simulink model "Car_State"  (R2023b)
settings: Solver=FixedStepAuto  StartTime=0.0  StopTime=10.0  RelTol=1e-3
libraries: simulink x5
settings Model: Creator=cspt  LastModifiedBy=joser
settings SolverCC: AlgebraicLoopSolver=TrustRegion
settings DataIOCC: SaveOutput=off  ReturnWorkspaceOutputs=off
settings OptimizationCC: DefaultParameterBehavior=Inlined
settings DebuggingCC: UnconnectedInputMsg=warning  UnconnectedOutputMsg=warning  UnconnectedLineMsg=warning  ArithmeticOperatorsInVariantConditions=warning
settings ModelReferenceCC: EnableRefExpFcnMdlSchedulingChecks=on
settings SFSimCC: SimUseLocalCustomCode=off  CustomCodeUndefinedFunction=UseInterfaceOnly
settings RTWCC: Description=INTECRIO Real-Time Target  SystemTargetFile=irt.tlc  TemplateMakefile=irt_default_tmf  RTWUseLocalCustomCode=off
settings STFCustomTargetCC: UtilityFuncGeneration=Shared location  MatFileLogging=on  GRTInterface=on  SystemTargetFile=irt.tlc
settings GRTTargetCC: UtilityFuncGeneration=Shared location  ParMdlRefBuildCompliant=off  CompOptLevelCompliant=off  ConcurrentExecutionCompliant=off  CombineOutputUpdateFcns=off  CPPClassGenCompliant=off  GRTInterface=on  UseToolchainInfoCompliant=off  GenerateASAP2=on

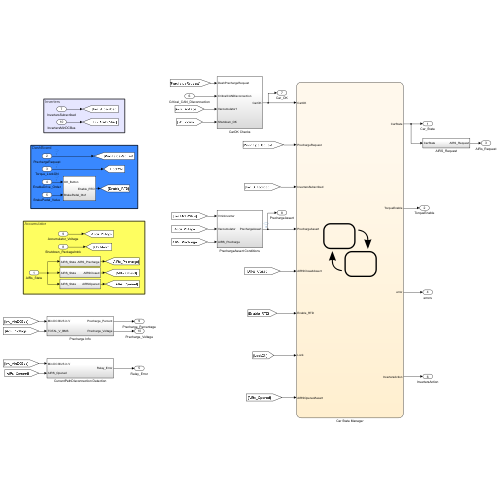
[thumbnail: Simulink's stored preview of the top-level diagram]
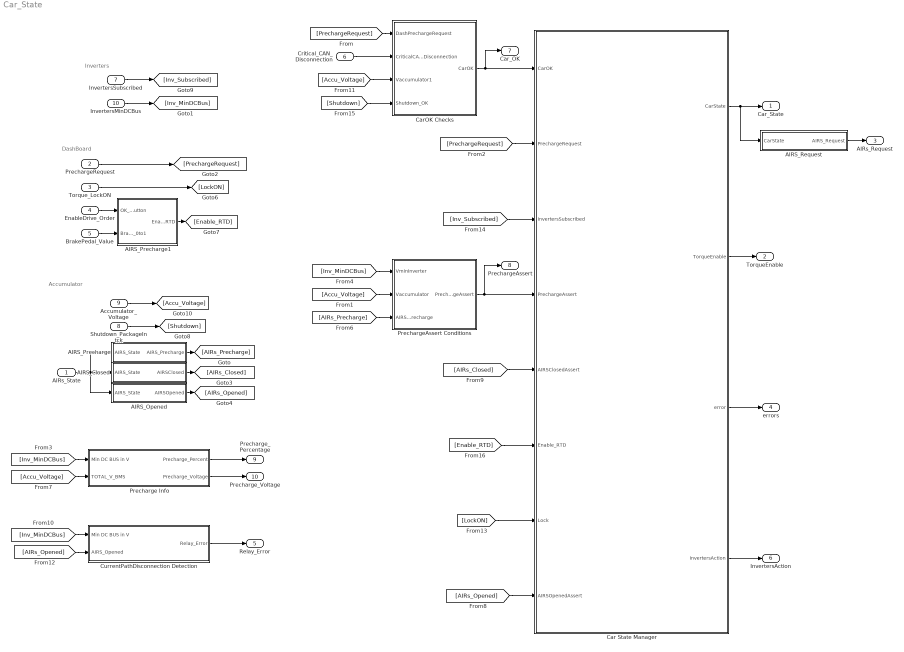
== system Car_State ==
  note: DashBoard
  note: Accumulator
  note: Inverters
  AIRs_State : Inport
  PrechargeRequest : Inport  Port=2
  Torque_LockON : Inport  Port=3
  EnableDrive_Order : Inport  Port=4
  BrakePedal_Value : Inport  Port=5
  Critical_CAN_Disconnection : Inport  Port=6
  InvertersSubscribed : Inport  Port=7
  Shutdown_PackageIntck : Inport  Port=8
  Accumulator_Voltage : Inport  Port=9  OutDataTypeStr=double  Unit=V
  InvertersMinDCBus : Inport  Port=10  Unit=V
  AIRS_Closed : Subsystem
  AIRS_Opened : Subsystem
  AIRS_Precharge : Subsystem
  AIRS_Precharge1 : Subsystem
  AIRS_Request : Subsystem
  Car State Manager : Stateflow chart  TreatAsAtomicUnit=on  SystemSampleTime=0.025
  CarOK Checks : Subsystem
  CurrentPathDisconnection Detection : Subsystem
  Precharge Info : Subsystem
  PrechargeAssert Conditions : Subsystem
  Car_State : Outport  VectorParamsAs1DForOutWhenUnconnected=off
  TorqueEnable : Outport  Port=2  VectorParamsAs1DForOutWhenUnconnected=off
  AIRs_Request : Outport  Port=3  VectorParamsAs1DForOutWhenUnconnected=off
  errors : Outport  Port=4  VectorParamsAs1DForOutWhenUnconnected=off
  Relay_Error : Outport  Port=5  VectorParamsAs1DForOutWhenUnconnected=off
  InvertersAction : Outport  Port=6  VectorParamsAs1DForOutWhenUnconnected=off
  Car_OK : Outport  Port=7  VectorParamsAs1DForOutWhenUnconnected=off
  PrechargeAssert : Outport  Port=8  VectorParamsAs1DForOutWhenUnconnected=off
  Precharge_Percentage : Outport  Port=9  VectorParamsAs1DForOutWhenUnconnected=off
  Precharge_Voltage : Outport  Port=10  VectorParamsAs1DForOutWhenUnconnected=off
  wires:
  CurrentPathDisconnection Detection/1(Relay_Error) -> Relay_Error/1
  Car State Manager/1(CarState) -> AIRS_Request/1(CarState), Car_State/1
  [PrechargeRequest] -> CarOK Checks/1(DashPrechargeRequest)
  AIRS_Request/1(AIRS_Request) -> AIRs_Request/1
  Car State Manager/4(InvertersAction) -> InvertersAction/1
  Car State Manager/2(TorqueEnable) -> TorqueEnable/1
  Car State Manager/3(error) -> errors/1
  CarOK Checks/1(CarOK) -> Car_OK/1, Car State Manager/1(CarOK)
  PrechargeRequest/1 -> [PrechargeRequest]
  AIRs_State/1 -> AIRS_Opened/1(AIRS_State), AIRS_Precharge/1(AIRS_State), AIRS_Closed/1(AIRS_State)
  Critical_CAN_Disconnection/1 -> CarOK Checks/2(CriticalCANDisconnection)
  Shutdown_PackageIntck/1 -> [Shutdown]
  [PrechargeRequest] -> Car State Manager/2(PrechargeRequest)
  [AIRs_Opened] -> Car State Manager/8(AIRSOpenedAssert)
  [AIRs_Closed] -> Car State Manager/5(AIRSClosedAssert)
  Torque_LockON/1 -> [LockON]
  EnableDrive_Order/1 -> AIRS_Precharge1/1(OK_Button)
  [Enable_RTD] -> Car State Manager/6(Enable_RTD)
  [LockON] -> Car State Manager/7(Lock)
  InvertersSubscribed/1 -> [Inv_Subscribed]
  [Inv_Subscribed] -> Car State Manager/3(InvertersSubscribed)
  [Shutdown] -> CarOK Checks/4(Shutdown_OK)
  PrechargeAssert Conditions/1(PrechargeAssert) -> Car State Manager/4(PrechargeAssert), PrechargeAssert/1
  [Inv_MinDCBus] -> Precharge Info/1(Min DC BUS in V)
  Precharge Info/1(Precharge_Percent) -> Precharge_Percentage/1
  Precharge Info/2(Precharge_Voltage) -> Precharge_Voltage/1
  [Inv_MinDCBus] -> CurrentPathDisconnection Detection/1(Min DC BUS in V)
  [AIRs_Opened] -> CurrentPathDisconnection Detection/2(AIRS_Opened)
  [Accu_Voltage] -> PrechargeAssert Conditions/2(Vaccumulator)
  [Inv_MinDCBus] -> PrechargeAssert Conditions/1(VminInverter)
  [AIRs_Precharge] -> PrechargeAssert Conditions/3(AIRS_Precharge)
  [Accu_Voltage] -> Precharge Info/2(TOTAL_V_BMS)
  Accumulator_Voltage/1 -> [Accu_Voltage]
  InvertersMinDCBus/1 -> [Inv_MinDCBus]
  AIRS_Closed/1(AIRSClosed) -> [AIRs_Closed]
  [Accu_Voltage] -> CarOK Checks/3(Vaccumulator1)
  AIRS_Precharge/1(AIRS_Precharge) -> [AIRs_Precharge]
  AIRS_Opened/1(AIRSOpened) -> [AIRs_Opened]
  BrakePedal_Value/1 -> AIRS_Precharge1/2(BrakePedal_0to1)
  AIRS_Precharge1/1(Enable_RTD) -> [Enable_RTD]

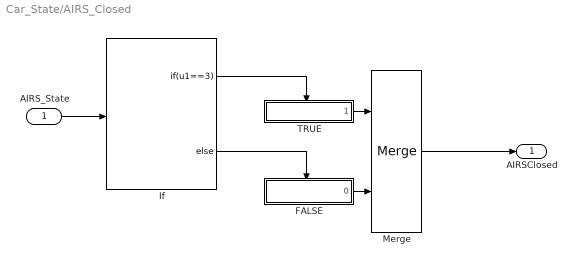
== system Car_State/AIRS_Closed ==
  AIRS_State : Inport
  FALSE : Subsystem  TreatAsAtomicUnit=on
  If : If  IfExpression=u1==3
  Merge : Merge
  TRUE : Subsystem  TreatAsAtomicUnit=on
  AIRSClosed : Outport  VectorParamsAs1DForOutWhenUnconnected=off
  wires:
  Merge/1 -> AIRSClosed/1
  FALSE/1(0) -> Merge/2
  If/2 -> FALSE/Action
  TRUE/1(1) -> Merge/1
  If/1 -> TRUE/Action
  AIRS_State/1 -> If/1

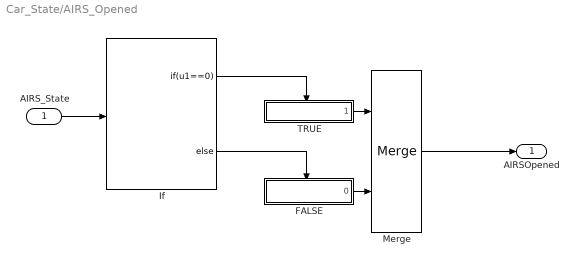
== system Car_State/AIRS_Opened ==
  AIRS_State : Inport
  FALSE : Subsystem  TreatAsAtomicUnit=on
  If : If  IfExpression=u1==0
  Merge : Merge
  TRUE : Subsystem  TreatAsAtomicUnit=on
  AIRSOpened : Outport  VectorParamsAs1DForOutWhenUnconnected=off
  wires:
  Merge/1 -> AIRSOpened/1
  FALSE/1(0) -> Merge/2
  If/2 -> FALSE/Action
  TRUE/1(1) -> Merge/1
  If/1 -> TRUE/Action
  AIRS_State/1 -> If/1

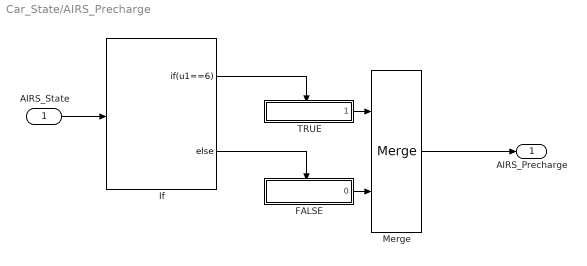
== system Car_State/AIRS_Precharge ==
  AIRS_State : Inport
  FALSE : Subsystem  TreatAsAtomicUnit=on
  If : If  IfExpression=u1==6
  Merge : Merge
  TRUE : Subsystem  TreatAsAtomicUnit=on
  AIRS_Precharge : Outport  VectorParamsAs1DForOutWhenUnconnected=off
  wires:
  Merge/1 -> AIRS_Precharge/1
  FALSE/1(0) -> Merge/2
  If/2 -> FALSE/Action
  TRUE/1(1) -> Merge/1
  If/1 -> TRUE/Action
  AIRS_State/1 -> If/1

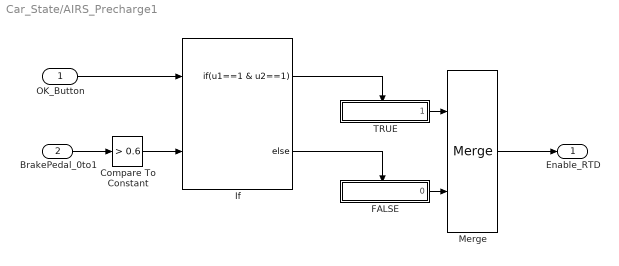
== system Car_State/AIRS_Precharge1 ==
  OK_Button : Inport
  BrakePedal_0to1 : Inport  Port=2
  Compare To Constant : simulink/Logic and Bit Operations/Compare To Constant  relop=>  const=0.6  OutDataTypeStr=boolean
  FALSE : Subsystem  TreatAsAtomicUnit=on
  If : If  NumInputs=2  IfExpression=u1==1 & u2==1
  Merge : Merge
  TRUE : Subsystem  TreatAsAtomicUnit=on
  Enable_RTD : Outport  VectorParamsAs1DForOutWhenUnconnected=off
  wires:
  Merge/1 -> Enable_RTD/1
  FALSE/1(0) -> Merge/2
  If/2 -> FALSE/Action
  TRUE/1(1) -> Merge/1
  If/1 -> TRUE/Action
  OK_Button/1 -> If/1
  BrakePedal_0to1/1 -> Compare To Constant/1
  Compare To Constant/1 -> If/2

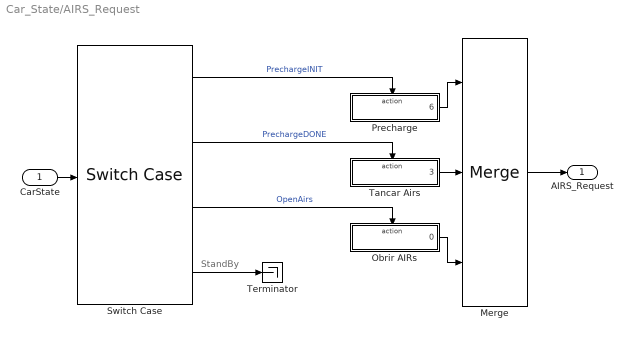
== system Car_State/AIRS_Request ==
  note: StandBy
  CarState : Inport
  Merge : Merge  Inputs=3
  Obrir AIRs : Subsystem  TreatAsAtomicUnit=on
  Precharge : Subsystem  TreatAsAtomicUnit=on
  Switch Case : SwitchCase  CaseConditions={6,9,21}
  Tancar Airs : Subsystem  TreatAsAtomicUnit=on
  Terminator : Terminator
  AIRS_Request : Outport  VectorParamsAs1DForOutWhenUnconnected=off
  wires:
  Merge/1 -> AIRS_Request/1
  Switch Case/2 -> Tancar Airs/Action  "PrechargeDONE"
  Switch Case/1 -> Precharge/Action  "PrechargeINIT"
  CarState/1 -> Switch Case/1
  Switch Case/3 -> Obrir AIRs/Action  "OpenAirs"
  Precharge/1(6) -> Merge/1
  Tancar Airs/1(3) -> Merge/2
  Obrir AIRs/1(0) -> Merge/3
  Switch Case/4 -> Terminator/1

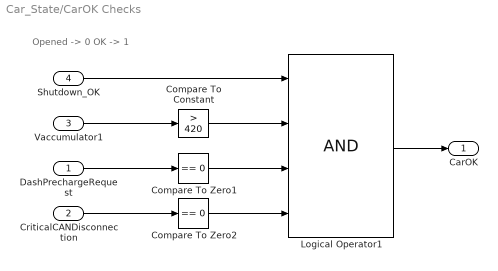
== system Car_State/CarOK Checks ==
  note: Opened -> 0
      | OK -> 1
  DashPrechargeRequest : Inport
  CriticalCANDisconnection : Inport  Port=2
  Vaccumulator1 : Inport  Port=3
  Shutdown_OK : Inport  Port=4
  Compare To Constant : simulink/Logic and Bit Operations/Compare To Constant  relop=>  const=420  OutDataTypeStr=boolean
  Compare To Zero1 : simulink/Logic and Bit Operations/Compare To Zero  relop===  OutDataTypeStr=boolean
  Compare To Zero2 : simulink/Logic and Bit Operations/Compare To Zero  relop===  OutDataTypeStr=boolean
  Logical Operator1 : Logic  Inputs=4  AllPortsSameDT=off  OutDataTypeStr=boolean
  CarOK : Outport  VectorParamsAs1DForOutWhenUnconnected=off
  wires:
  Logical Operator1/1 -> CarOK/1
  DashPrechargeRequest/1 -> Compare To Zero1/1
  Compare To Zero1/1 -> Logical Operator1/3
  CriticalCANDisconnection/1 -> Compare To Zero2/1
  Compare To Zero2/1 -> Logical Operator1/4
  Shutdown_OK/1 -> Logical Operator1/1
  Vaccumulator1/1 -> Compare To Constant/1
  Compare To Constant/1 -> Logical Operator1/2

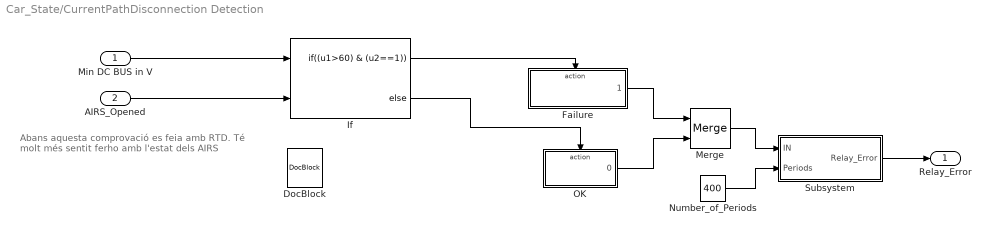
== system Car_State/CurrentPathDisconnection Detection ==
  note: Abans aquesta comprovació es feia amb RTD.
      | Té molt més sentit ferho amb l'estat dels AIRS
  Min DC BUS in V : Inport
  AIRS_Opened : Inport  Port=2
  DocBlock : simulink/Model-Wide Utilities/DocBlock  DocumentType=Text
      content=|
      | In case the Inverters DC Bus is higher than 60V & the AIRs are opened, then
      | the Relays could be welded.
      |
      | This subsystem checks if those conditions have been persistent for more
      | than 10 sec: Number of periods = 10sec / 0.025sec = 400 periods
      | 10sec is the maximum time for the Bus to be discharged. If the condition
      | persists for more than 10sec, that's an error (for example, Relays welded)
      |
      | SIGNAL JUST FOR CHECK ON THE CANoe, NO REAL APPLICATION.
  Failure : Subsystem  TreatAsAtomicUnit=on
  If : If  NumInputs=2  IfExpression=(u1>60) & (u2==1)
  Merge : Merge
  Number_of_Periods : Constant  Value=400
  OK : Subsystem  TreatAsAtomicUnit=on
  Subsystem : Subsystem
  Relay_Error : Outport  VectorParamsAs1DForOutWhenUnconnected=off
  wires:
  OK/1(0) -> Merge/2
  Merge/1 -> Subsystem/1(IN)
  If/2 -> OK/Action
  If/1 -> Failure/Action
  Failure/1("1 ") -> Merge/1
  Min DC BUS in V/1 -> If/1
  AIRS_Opened/1 -> If/2
  Subsystem/1(Relay_Error) -> Relay_Error/1
  Number_of_Periods/1 -> Subsystem/2(Periods)

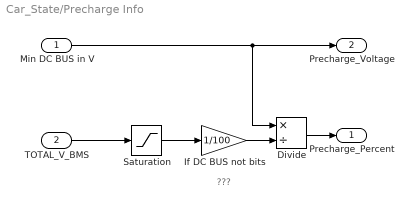
== system Car_State/Precharge Info ==
  note: ???
  Min DC BUS in V : Inport
  TOTAL_V_BMS : Inport  Port=2
  Divide : Product  Inputs=*/
  If DC BUS not bits : Gain  Gain=1/100
  Saturation : Saturate  UpperLimit=600  LowerLimit=400
  Precharge_Percent : Outport  VectorParamsAs1DForOutWhenUnconnected=off
  Precharge_Voltage : Outport  Port=2  VectorParamsAs1DForOutWhenUnconnected=off
  wires:
  Min DC BUS in V/1 -> Precharge_Voltage/1, Divide/1
  Saturation/1 -> If DC BUS not bits/1
  Divide/1 -> Precharge_Percent/1
  If DC BUS not bits/1 -> Divide/2
  TOTAL_V_BMS/1 -> Saturation/1

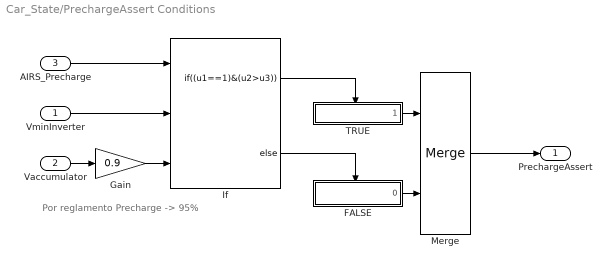
== system Car_State/PrechargeAssert Conditions ==
  note: Por reglamento Precharge -> 95%
  VminInverter : Inport
  Vaccumulator : Inport  Port=2
  AIRS_Precharge : Inport  Port=3
  FALSE : Subsystem  TreatAsAtomicUnit=on
  Gain : Gain  Gain=0.9  OutDataTypeStr=Inherit: Same as input
  If : If  NumInputs=3  IfExpression=(u1==1)&(u2>u3)
  Merge : Merge
  TRUE : Subsystem  TreatAsAtomicUnit=on
  PrechargeAssert : Outport  VectorParamsAs1DForOutWhenUnconnected=off
  wires:
  If/2 -> FALSE/Action
  FALSE/1(0) -> Merge/2
  TRUE/1(1) -> Merge/1
  If/1 -> TRUE/Action
  Merge/1 -> PrechargeAssert/1
  Vaccumulator/1 -> Gain/1
  Gain/1 -> If/3
  AIRS_Precharge/1 -> If/1
  VminInverter/1 -> If/2

== system Car_State/AIRS_Closed/FALSE ==
  Action Port : ActionPort  ActionPortLabel=else
  Constant : Constant  Value=0
  0 : Outport  VectorParamsAs1DForOutWhenUnconnected=off
  wires:
  Constant/1 -> 0/1

== system Car_State/AIRS_Closed/TRUE ==
  Action Port : ActionPort  ActionPortLabel=if(u1==3)
  Constant : Constant
  1 : Outport  VectorParamsAs1DForOutWhenUnconnected=off
  wires:
  Constant/1 -> 1/1

== system Car_State/AIRS_Opened/FALSE ==
  Action Port : ActionPort  ActionPortLabel=else
  Constant : Constant  Value=0
  0 : Outport  VectorParamsAs1DForOutWhenUnconnected=off
  wires:
  Constant/1 -> 0/1

== system Car_State/AIRS_Opened/TRUE ==
  Action Port : ActionPort  ActionPortLabel=if(u1==0)
  Constant : Constant
  1 : Outport  VectorParamsAs1DForOutWhenUnconnected=off
  wires:
  Constant/1 -> 1/1

== system Car_State/AIRS_Precharge/FALSE ==
  Action Port : ActionPort  ActionPortLabel=else
  Constant : Constant  Value=0
  0 : Outport  VectorParamsAs1DForOutWhenUnconnected=off
  wires:
  Constant/1 -> 0/1

== system Car_State/AIRS_Precharge/TRUE ==
  Action Port : ActionPort  ActionPortLabel=if(u1==6)
  Constant : Constant
  1 : Outport  VectorParamsAs1DForOutWhenUnconnected=off
  wires:
  Constant/1 -> 1/1

== system Car_State/AIRS_Precharge1/FALSE ==
  Action Port : ActionPort  ActionPortLabel=else
  Constant : Constant  Value=0
  0 : Outport  VectorParamsAs1DForOutWhenUnconnected=off
  wires:
  Constant/1 -> 0/1

== system Car_State/AIRS_Precharge1/TRUE ==
  Action Port : ActionPort  ActionPortLabel=if(u1==1 & u2==1)
  Constant : Constant
  1 : Outport  VectorParamsAs1DForOutWhenUnconnected=off
  wires:
  Constant/1 -> 1/1

== system Car_State/AIRS_Request/Obrir AIRs ==
  Action Port : ActionPort  ActionPortLabel=case [ 21 ]:
  Constant : Constant  Value=0
  0 : Outport  VectorParamsAs1DForOutWhenUnconnected=off
  wires:
  Constant/1 -> 0/1

== system Car_State/AIRS_Request/Precharge ==
  Action Port : ActionPort  ActionPortLabel=case [ 6 ]:
  Constant : Constant  Value=6
  6 : Outport  VectorParamsAs1DForOutWhenUnconnected=off
  wires:
  Constant/1 -> 6/1

== system Car_State/AIRS_Request/Tancar Airs ==
  Action Port : ActionPort  ActionPortLabel=case [ 9 ]:
  Constant : Constant  Value=3
  3 : Outport  VectorParamsAs1DForOutWhenUnconnected=off
  wires:
  Constant/1 -> 3/1

== system Car_State/CurrentPathDisconnection Detection/Failure ==
  Action Port : ActionPort  ActionPortLabel=if((u1<60)&(u2==1))
  Constant : Constant
  "1 " : Outport  VectorParamsAs1DForOutWhenUnconnected=off
  wires:
  Constant/1 -> "1 "/1

== system Car_State/CurrentPathDisconnection Detection/OK ==
  Action Port : ActionPort  ActionPortLabel=else
  Constant : Constant  Value=0
  0 : Outport
  wires:
  Constant/1 -> 0/1

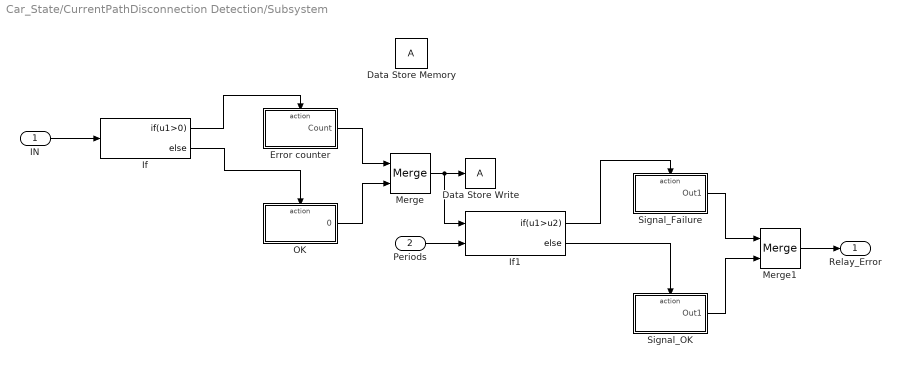
== system Car_State/CurrentPathDisconnection Detection/Subsystem ==
  IN : Inport
  Periods : Inport  Port=2
  Data Store Memory : DataStoreMemory  WriteAfterWriteMsg=warning  ShowAdditionalParam=off
  Data Store Write : DataStoreWrite  IndexOptions=Index vector (dialog)  Indices=1  OutputSizes=1
  Error counter : Subsystem  TreatAsAtomicUnit=on
  If : If  IfExpression=u1>0
  If1 : If  NumInputs=2  IfExpression=u1>u2
  Merge : Merge
  Merge1 : Merge
  OK : Subsystem  TreatAsAtomicUnit=on
  Signal_Failure : Subsystem  TreatAsAtomicUnit=on
  Signal_OK : Subsystem  TreatAsAtomicUnit=on
  Relay_Error : Outport  VectorParamsAs1DForOutWhenUnconnected=off
  wires:
  Periods/1 -> If1/2
  Signal_Failure/1(Out1) -> Merge1/1
  If1/2 -> Signal_OK/Action
  Signal_OK/1(Out1) -> Merge1/2
  If1/1 -> Signal_Failure/Action
  Merge/1 -> Data Store Write/1, If1/1
  OK/1("0 ") -> Merge/2
  If/1 -> Error counter/Action
  Error counter/1("Count ") -> Merge/1
  Merge1/1 -> Relay_Error/1
  If/2 -> OK/Action
  IN/1 -> If/1

== system Car_State/PrechargeAssert Conditions/FALSE ==
  Action Port : ActionPort  ActionPortLabel=else
  Constant : Constant  Value=0
  0 : Outport  VectorParamsAs1DForOutWhenUnconnected=off
  wires:
  Constant/1 -> 0/1

== system Car_State/PrechargeAssert Conditions/TRUE ==
  Action Port : ActionPort  ActionPortLabel=if((u1==1)&(u2>u3))
  Constant : Constant
  1 : Outport  VectorParamsAs1DForOutWhenUnconnected=off
  wires:
  Constant/1 -> 1/1

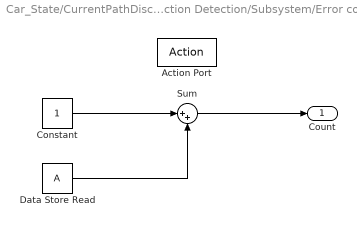
== system Car_State/CurrentPathDisconnection Detection/Subsystem/Error counter ==
  Action Port : ActionPort  ActionPortLabel=if((u1>0))
  Constant : Constant
  Data Store Read : DataStoreRead  IndexOptions=Index vector (dialog)  Indices=1  OutputSizes=1
  Sum : Sum  Inputs=|++
  "Count " : Outport  VectorParamsAs1DForOutWhenUnconnected=off
  wires:
  Constant/1 -> Sum/1
  Data Store Read/1 -> Sum/2
  Sum/1 -> "Count "/1

== system Car_State/CurrentPathDisconnection Detection/Subsystem/OK ==
  Action Port : ActionPort  ActionPortLabel=else
  Constant : Constant  Value=0
  "0 " : Outport  VectorParamsAs1DForOutWhenUnconnected=off
  wires:
  Constant/1 -> "0 "/1

== system Car_State/CurrentPathDisconnection Detection/Subsystem/Signal_Failure ==
  Action Port : ActionPort  ActionPortLabel=if(u1>u2)
  Constant : Constant
  Out1 : Outport  VectorParamsAs1DForOutWhenUnconnected=off
  wires:
  Constant/1 -> Out1/1

== system Car_State/CurrentPathDisconnection Detection/Subsystem/Signal_OK ==
  Action Port : ActionPort  ActionPortLabel=else
  Constant : Constant  Value=0
  Out1 : Outport  VectorParamsAs1DForOutWhenUnconnected=off
  wires:
  Constant/1 -> Out1/1

== stateflow chart Car_State/Car State Manager ==
  state SAFESTATE [group]
    state Init
      entry: CarState=0;
      TorqueEnable=0;
      InvertersAction=20;
    state Standby
      entry: CarState=3;
      TorqueEnable=0;
      InvertersAction=11;
    (default) -> Init : {error=0}
    Standby -> Init [order 2] : [CarOK==0]
    Init -> Standby : [CarOK==1 & after(1, sec)]
  state STOP [group]
    state OpenAirs
      entry: CarState=21;
      InvertersAction=20;
  note: Inverter Actions that can be commanded to the inverters:
      |
      | Unsubscribe -> 10
      | Subscribe -> 11
      | DisableDrive -> 20
      | EnableDrive -> 21
      | TorqueCommand -> 30
      |
      |
      | El CarState -> 13 si se ha elegido el Custom Mode
  state PRECHARGE [group]
    state PrechargeINIT
      entry: CarState=6;
      TorqueEnable=0;
      InvertersAction=20;
    state PrechargeDONE
      entry: CarState=9;
      TorqueEnable=0;
      InvertersAction=20;
    PrechargeINIT -> PrechargeDONE [order 1] : [PrechargeAssert==1 & after(2500,msec)]
  state ACTIVE [group]
    state TSActive
      entry: CarState=12;
      TorqueEnable=0;
      InvertersAction=20;
    state EnableInverters
      entry: CarState=14;
      TorqueEnable=0;
      InvertersAction=21;
    state RTD
      entry: CarState=15;
      TorqueEnable=1;
      InvertersAction=30;
    state Locked
      entry: CarState=13;
      TorqueEnable=0;
      InvertersAction=20;
    EnableInverters -> RTD [order 1] : [after(2,sec)]
    TSActive -> EnableInverters [order 1] : [Enable_RTD==1]
    TSActive -> Locked [order 3] : [Lock==1]
    Locked -> EnableInverters [order 1] : [Enable_RTD==1 & Lock==0]
  OpenAirs -> Init : [AIRSOpenedAssert==1 & after(1,sec)]
  Standby -> PrechargeINIT [order 1] : [PrechargeRequest==1 & InvertersSubscribed==1]
  PrechargeINIT -> OpenAirs [order 2] : after(10,sec)
      | {error=6}
  PrechargeDONE -> OpenAirs [order 3] : [CarOK==0]
  PrechargeDONE -> OpenAirs [order 1] : after(2,sec)
      | {error=9}
  TSActive -> OpenAirs [order 2] : [CarOK==0]
  Locked -> OpenAirs [order 2] : [CarOK==0]
  EnableInverters -> OpenAirs [order 2] : [CarOK==0]
  RTD -> OpenAirs : [CarOK==0]
  PrechargeDONE -> TSActive [order 2] : [AIRSClosedAssert==1 & after(100,msec)]
  data: CarOK input; PrechargeRequest input; InvertersSubscribed input; CarState output double; PrechargeAssert input; AIRSClosedAssert input; Enable_RTD input; Lock input double; AIRSOpenedAssert input; TorqueEnable output double; error output double; InvertersAction output double
